simulink model "TestAsset14"  (R2018b)
settings: Solver=ode45  StartTime=0.0  StopTime=4  RelTol=1e-3  EnableMultiTasking=on
undefined symbols (not defined in the file): c1, c2, c3, c4, c5, c6, DiscIntNeverNeededParam, fdesignblkfcn, gcbh, Hydride, Metal, Nickel
libraries: powerlib x63, powerlib_extras x26, powerlib_meascontrol x25, simulink x5, simulink_extras x2, electricdrivelib x1
(part 2 of 3)

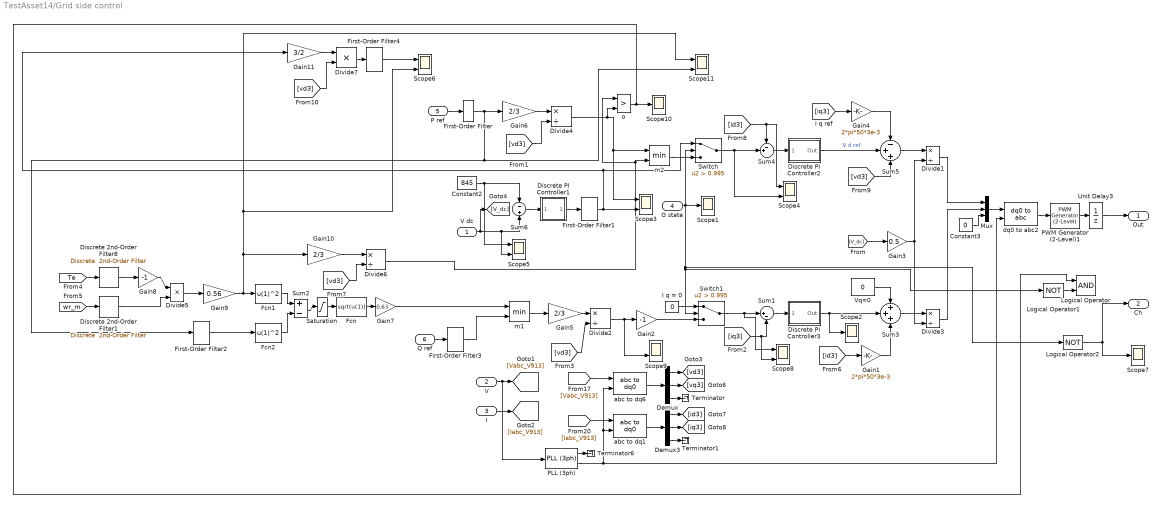
== system TestAsset14/Grid side control ==
  V dc : Inport
  V : Inport  Port=2
  I : Inport  Port=3
  G state : Inport  Port=4
  P ref : Inport  Port=5
  Q ref : Inport  Port=6
  Constant2 : Constant  Value=845
  Constant3 : Constant  Value=0
  Demux : Demux  Outputs=3
  Demux3 : Demux  Outputs=3
  Discrete PI Controller1 : Subsystem  DialogController=POWERSYS.PowerSysDialog  mask(Discrete PI Controller){Kp=10, Ki=60, Par_Limits=[500 -500], Init=0, Ts=20e-6}
      mask prompts: Kp "Proportional gain (Kp):"; Ki "Integral gain (Ki):"; Par_Limits "Output limits: [ Upper   Lower ]"; Init "Output initial value:"; Ts "Sample time:"
      mask help: This block implements a discrete PI controller.
      mask init:
      | UpperLimit=Par_Limits(1);
      | LowerLimit=Par_Limits(2);
      | power_initmask();
      mask Display: disp('PI');
  Discrete PI Controller2 : Subsystem  DialogController=POWERSYS.PowerSysDialog  mask(Discrete PI Controller){Kp=16, Ki=160, Par_Limits=[400 -400], Init=0, Ts=20e-6}
      mask prompts: Kp "Proportional gain (Kp):"; Ki "Integral gain (Ki):"; Par_Limits "Output limits: [ Upper   Lower ]"; Init "Output initial value:"; Ts "Sample time:"
      mask help: This block implements a discrete PI controller.
      mask init:
      | UpperLimit=Par_Limits(1);
      | LowerLimit=Par_Limits(2);
      | power_initmask();
      mask Display: disp('PI');
  Discrete PI Controller3 : Subsystem  DialogController=POWERSYS.PowerSysDialog  mask(Discrete PI Controller){Kp=16, Ki=160, Par_Limits=[400 -400], Init=0, Ts=20e-6}
      mask prompts: Kp "Proportional gain (Kp):"; Ki "Integral gain (Ki):"; Par_Limits "Output limits: [ Upper   Lower ]"; Init "Output initial value:"; Ts "Sample time:"
      mask help: This block implements a discrete PI controller.
      mask init:
      | UpperLimit=Par_Limits(1);
      | LowerLimit=Par_Limits(2);
      | power_initmask();
      mask Display: disp('PI');
  Discrete 2nd-Order Filter1 : powerlib_extras/Discrete  Control Blocks/Discrete  2nd-Order Filter  FilterType=Lowpass  Fo=50  Zeta=0.73  Ts=20e-6  Initialize=on  Vac_Init=[0.8 -25 60]*0  Vdc_Init=-183.8  PlotResponse=off  param1=[1 500 1]
  Discrete 2nd-Order Filter8 : powerlib_extras/Discrete  Control Blocks/Discrete  2nd-Order Filter  FilterType=Lowpass  Fo=50  Zeta=0.73  Ts=20e-6  Initialize=on  Vac_Init=[0.8 -25 60]*0  Vdc_Init=-183.8  PlotResponse=off  param1=[1 500 1]
  Divide{1..4,6} (5 alike) : Product  Inputs=*/
  Divide5 : Product  Inputs=**
  Divide7 : Product  Inputs=**
  Fcn : Fcn  Expr=sqrt(u(1))
  Fcn1 : Fcn  Expr=u(1)^2  SampleTime=20e-6
  Fcn2 : Fcn  Expr=u(1)^2  SampleTime=20e-6
  First-Order Filter{,1..4} (5 alike) : powerlib_meascontrol/Filters/First-Order Filter  FilterType=Lowpass  Tc=10e-3  Ts=20e-6  Initialize=on  Vac_Init=[0, 0, 60]  Vdc_Init=0  PlotResponse=off  FreqRange="[0,  200,  1]"
  Gain1 : Gain  Gain=2*pi*50*3e-3
  Gain10 : Gain  Gain=2/3
  Gain11 : Gain  Gain=3/2
  Gain2 : Gain  Gain=-1
  Gain3 : Gain  Gain=0.5
  Gain4 : Gain  Gain=2*pi*50*3e-3
  Gain5 : Gain  Gain=2/3
  Gain6 : Gain  Gain=2/3
  Gain7 : Gain  Gain=0.63
  Gain8 : Gain  Gain=-1
  Gain9 : Gain  Gain=0.56
  I q = 0 : Constant  Value=0
  Logical Operator : Logic  AllPortsSameDT=off  OutDataTypeStr=boolean  SampleTime=20e-6
  Logical Operator1 : Logic  Operator=NOT  AllPortsSameDT=off  OutDataTypeStr=boolean  SampleTime=20e-6
  Logical Operator2 : Logic  Operator=NOT  AllPortsSameDT=off  OutDataTypeStr=boolean  SampleTime=20e-6
  Mux : Mux  Inputs=3
  PLL (3ph) : powerlib_meascontrol/PLL/PLL (3ph)  Fmin=45  Par_Init=[0, 60]  ParK=[180, 3200, 1]  TcD=1e-4  MaxRateChangeFreq=12  FilterCutOffFreq=25  Ts=20e-6  AGC=on
  PWM Generator (2-Level)1 : powerlib_meascontrol/Pulse & Signal Generators/PWM Generator (2-Level)  ModulatorType=Three-phase bridge (6 pulses)  ModulatorMode=Unsynchronized  Fc=2000  Pc=90  nF=27  MinMax="[ -1  1 ]"  SamplingTechnique=Natural  ModulatingSignals=off  m=0.8  Freq=60  Phase=0  Ts=20e-6  ShowCarrierOutport=off
  Saturation : Saturate  UpperLimit=inf  LowerLimit=0
  Scope{1..2,7,10} (4 alike) : Scope
  Scope{3..6,8..9,11} (7 alike) : Scope  NumInputPorts=2
  Sum1 : Sum  Inputs=|+-
  Sum2 : Sum  Inputs=+-
  Sum3 : Sum  Inputs=+++
  Sum4 : Sum  Inputs=-+|
  Sum5 : Sum  Inputs=-++
  Sum6 : Sum  Inputs=-+
  Switch : Switch  Criteria=u2 > Threshold  Threshold=0.995
  Switch1 : Switch  Criteria=u2 > Threshold  Threshold=0.995
  Terminator : Terminator
  Terminator1 : Terminator
  Terminator6 : Terminator
  Unit Delay3 : UnitDelay  SampleTime=2e-05  HasFrameUpgradeWarning=on
  Vq=0 : Constant  Value=0
  abc to dq1 : powerlib_meascontrol/Transformations/abc to dq0  Alignment=90 degrees behind phase A axis
  abc to dq6 : powerlib_meascontrol/Transformations/abc to dq0  Alignment=90 degrees behind phase A axis
  dq0 to abc2 : powerlib_meascontrol/Transformations/dq0 to abc  Alignment=90 degrees behind phase A axis
  m1 : MinMax  Inputs=2  SampleTime=20e-6
  m2 : MinMax  Inputs=2  SampleTime=20e-6
  o : RelationalOperator  Operator=>  OutDataTypeStr=boolean  RndMeth=Nearest
  Out : Outport
  Ch : Outport  Port=2
  wires:
  abc to dq6/1 -> Demux/1
  Demux/1 -> [vd3]
  Demux/2 -> [vq3]
  abc to dq1/1 -> Demux3/1
  Demux3/1 -> [id3]
  Demux3/2 -> [iq3]
  [iq3] -> Scope8/2, Sum1/2
  Sum1/1 -> Discrete PI Controller3/1(Error)
  Discrete PI Controller3/1(Out) -> Scope2/1, Sum3/2
  Gain1/1 -> Sum3/3
  [id3] -> Gain1/1
  Sum3/1 -> Divide3/1
  Mux/1 -> dq0 to abc2/1
  [Vabc_V913] -> abc to dq6/1
  [Iabc_V913] -> abc to dq1/1
  dq0 to abc2/1 -> PWM Generator (2-Level)1/1
  Constant3/1 -> Mux/3
  PLL (3ph)/2 -> dq0 to abc2/2, abc to dq1/2, abc to dq6/2
  V/1 -> PLL (3ph)/1, [Vabc_V913]
  Discrete PI Controller2/1(Out) -> Sum5/2  "V d ref"
  [vd3] -> Sum5/3
  Sum4/1 -> Discrete PI Controller2/1(Error)
  Gain4/1 -> Sum5/1
  Sum6/1 -> Discrete PI Controller1/1(Error)
  Sum5/1 -> Divide1/1
  I/1 -> [Iabc_V913]
  [iq3] -> Gain4/1
  Demux/3 -> Terminator/1
  Demux3/3 -> Terminator1/1
  Vq=0/1 -> Sum3/1
  Divide1/1 -> Mux/1
  Divide3/1 -> Mux/2
  Gain3/1 -> Divide1/2, Divide3/2
  [V_dc] -> Gain3/1
  PLL (3ph)/1 -> Terminator6/1
  [id3] -> Scope4/1, Sum4/1
  Switch1/1 -> Scope8/1, Sum1/1
  G state/1 -> Switch/2, Scope1/1, Logical Operator2/1, Logical Operator1/1, Switch1/2
  Divide4/1 -> o/2, m2/1, Scope3/1
  Switch/1 -> Scope4/2, Sum4/2
  [vd3] -> Divide4/2
  Gain6/1 -> Divide4/1
  m2/1 -> Switch/3
  Discrete PI Controller1/1(Out) -> First-Order Filter1/1
  I q = 0/1 -> Switch1/1
  [vd3] -> Divide2/2
  Gain5/1 -> Divide2/1
  Saturation/1 -> Fcn/1
  PWM Generator (2-Level)1/1 -> Unit Delay3/1
  Unit Delay3/1 -> Out/1
  Logical Operator2/1 -> Ch/1, Scope7/1
  o/1 -> Scope10/1, Logical Operator/1
  Logical Operator1/1 -> Logical Operator/2
  Gain2/1 -> Switch1/3
  Gain8/1 -> Divide5/1
  Discrete 2nd-Order Filter1/1 -> Divide5/2
  Divide5/1 -> Gain9/1
  V dc/1 -> Scope5/2, Sum6/2, [V_dc]
  Discrete 2nd-Order Filter8/1 -> Gain8/1
  [Te] -> Discrete 2nd-Order Filter8/1
  Gain9/1 -> Scope11/1, Scope6/2, Gain10/1, Fcn1/1
  [wr_m] -> Discrete 2nd-Order Filter1/1
  Fcn1/1 -> Sum2/1
  Fcn2/1 -> Sum2/2
  Sum2/1 -> Saturation/1
  Divide2/1 -> Scope9/2, Gain2/1
  First-Order Filter2/1 -> Fcn2/1
  First-Order Filter3/1 -> m1/2
  Q ref/1 -> First-Order Filter3/1
  Gain7/1 -> m1/1
  Fcn/1 -> Gain7/1
  Constant2/1 -> Sum6/1, Scope5/1
  [vd3] -> Divide7/2
  Gain11/1 -> Divide7/1
  Divide7/1 -> First-Order Filter4/1
  First-Order Filter4/1 -> Scope6/1
  First-Order Filter1/1 -> Gain11/1, Switch/1, Scope3/2
  m1/1 -> Gain5/1
  P ref/1 -> First-Order Filter/1
  First-Order Filter/1 -> Scope11/2, First-Order Filter2/1, Gain6/1
  Gain10/1 -> Divide6/1
  [vd3] -> Divide6/2
  Divide6/1 -> o/1, m2/2

== system TestAsset14/LC Filter ==
  "2 mH " : powerlib/Elements/Three-Phase Series RLC Branch  LConnTagsString=A|B|C  RConnTagsString=A|B|C  BranchType=L  Resistance=1.0  Inductance=3e-3  Capacitance=1.0  Measurements=None
  Ground : powerlib/Elements/Ground  LConnTagsString=a
  Ground1 : powerlib/Elements/Ground  LConnTagsString=a
  Ground2 : powerlib/Elements/Ground  LConnTagsString=a
  Three-Phase Series RLC Branch : powerlib/Elements/Three-Phase Series RLC Branch  LConnTagsString=A|B|C  RConnTagsString=A|B|C  BranchType=C  Resistance=.1  Inductance=1e-3  Capacitance=100e-6  Measurements=None
  A : PMIOPort  Side=Left
  B : PMIOPort  Port=2  Side=Left
  C : PMIOPort  Port=3  Side=Left
  "A " : PMIOPort  Port=4  Side=Right
  "B " : PMIOPort  Port=5  Side=Right
  "C " : PMIOPort  Port=6  Side=Right
  connections:
  B/RConn1 -- "2 mH "/LConn2
  A/RConn1 -- "2 mH "/LConn1
  C/RConn1 -- "2 mH "/LConn3
  "2 mH "/RConn1 -- "A "/RConn1 -- Three-Phase Series RLC Branch/LConn1
  "2 mH "/RConn2 -- "B "/RConn1 -- Three-Phase Series RLC Branch/LConn2
  "2 mH "/RConn3 -- "C "/RConn1 -- Three-Phase Series RLC Branch/LConn3
  Ground/LConn1 -- Three-Phase Series RLC Branch/RConn1
  Ground1/LConn1 -- Three-Phase Series RLC Branch/RConn2
  Ground2/LConn1 -- Three-Phase Series RLC Branch/RConn3

== system TestAsset14/LC Filter1 ==
  "2 mH " : powerlib/Elements/Three-Phase Series RLC Branch  LConnTagsString=A|B|C  RConnTagsString=A|B|C  BranchType=L  Resistance=0  Inductance=3e-3  Capacitance=inf  Measurements=None
  3 kvar : powerlib/Elements/Three-Phase Series RLC Load  LConnTagsString=A|B|C  Configuration=Y (grounded)  NominalVoltage=480  NominalFrequency=50  ActivePower=0  InductivePower=0  CapacitivePower=3e3  Measurements=None  LoadType=constant Z
  A : PMIOPort  Side=Left
  B : PMIOPort  Port=2  Side=Left
  C : PMIOPort  Port=3  Side=Left
  "A " : PMIOPort  Port=4  Side=Right
  "B " : PMIOPort  Port=5  Side=Right
  "C " : PMIOPort  Port=6  Side=Right
  connections:
  C/RConn1 -- "2 mH "/LConn3
  "2 mH "/LConn2 -- B/RConn1
  "2 mH "/LConn1 -- A/RConn1
  "A "/RConn1 -- 3 kvar/LConn1 -- "2 mH "/RConn1
  3 kvar/LConn3 -- "2 mH "/RConn3 -- "C "/RConn1
  3 kvar/LConn2 -- "2 mH "/RConn2 -- "B "/RConn1

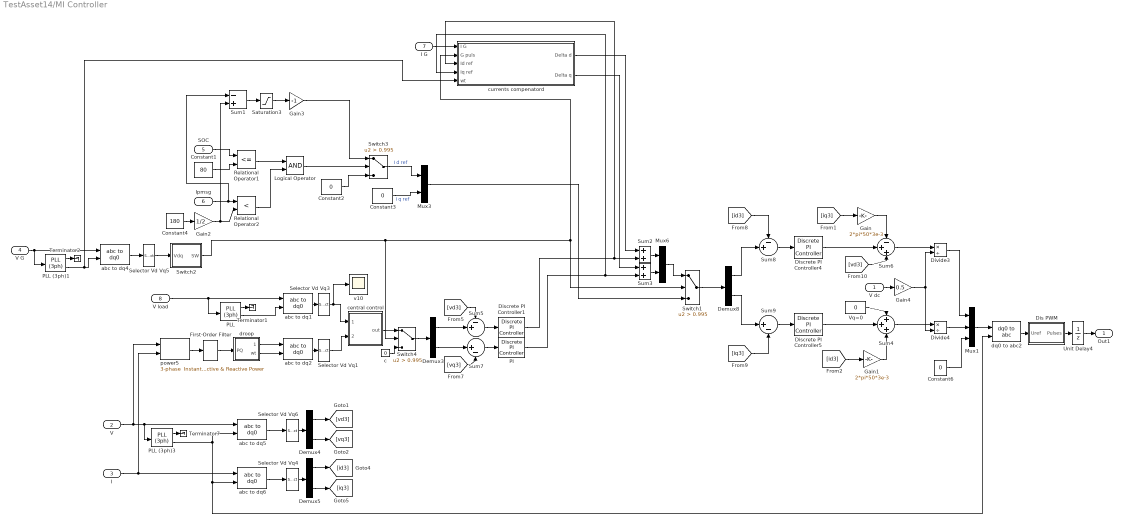
== system TestAsset14/MI Controller ==
  V dc : Inport
  V : Inport  Port=2
  I : Inport  Port=3
  V G : Inport  Port=4
  SOC : Inport  Port=5
  Ipmsg : Inport  Port=6
  I G : Inport  Port=7
  V load : Inport  Port=8
  Constant1 : Constant  Value=80
  Constant2 : Constant  Value=0
  Constant3 : Constant  Value=0
  Constant4 : Constant  Value=180
  Constant6 : Constant  Value=0
  Demux{3..5,8} (4 alike) : Demux  Outputs=2
  Dis PWM : Subsystem  AncestorBlock=|  DialogController=POWERSYS.PowerSysDialog  mask(Discrete PWM Generator){GeneratorMode=3-arm  bridge (6 pulses), Fc=4000, Ts=20e-6, Internal=off, mIndex=0.4, Freq=60, Phase=0}
      | powerlib_extras/Discrete 
      | Control Blocks/Discrete
      | PWM Generator
      mask prompts: GeneratorMode "Generator Mode"; Fc "Carrier frequency (Hz):"; Ts "Sample time:"; Internal "Internal generation of modulating signal(s)"; mIndex "Modulation index  (0<m<1) :"; Freq "Frequency of output voltage (Hz)"; Phase "Phase of output voltage (degrees)"
      mask help:
      | This discrete block generates pulses for carrier-based PWM (Pulse Width Modulation), self-commutated IGBTs,GTOs or FETs bridges.
      |
      | Depending on the number of bridge arms selected in the "Generator Mode" parameter, the block can be used either for single-phase or three-phase PWM control.
      mask init:
      | powericon('psbcallbacks',gcb,'Discrete PWM Generator');
      | if Freq==0
      |     Phase=90;
      | end
      | switch GeneratorMode
      | case 1,
      |     Internal_Phase=0;
      |    Signal_PortWidth=1;
      |    Select1_Elements=[1 2];
      |    Select1_PortWidth=2;
      |    Select3_Elements=[1 2];
      |    Select3_PortWidth=4;
      | case 2,
      |     Internal_Phase=0;
      |     Signal_PortWidth=1;
      |     Select1_Elements=[1 2];
      |     Select1_PortWidth=2;
      |     Select3_Elements=[1 2 3 4];
      |     Select3_PortWidth=4;
      | case 3,
      |     Internal_Phase=[0 -2*pi/3 2*pi/3];
      |     Signal_PortWidth=3;
      |     Select1_Elements=[1 4 2 5 3 6];
      |     Select1_PortWidth=6;
      |    Select3_Elements=[1 2 3 4 5 6];
      |    Select3_PortWidth=12;
      | case 4,
      |     Internal_Phase=[0 -2*pi/3 2*pi/3];
      |     Signal_PortWidth=3;
      |     Select1_Elements=[1 4 2 5 3 6];
      |     Select1_PortWidth=6;
      |    Select3_Elements=[1 2 3 4 5 6 7 8 9 10 11 12];
      |    Select3_PortWidth=12;
      | end
      | power_initmask();
      mask Help:
      | The output pulses are a vector (with values=0 or 1). Depending on the selected "Generator Mode", the output vector contains:
      | For a 1-arm  bridge: Two pulses. Pulse 1 is for the upper switch and pulse 2 is for the lower switch.
      | For a 2-arm  bridge: Four pulses. Pulses 1 and 3 are respectively for the upper switches of the first and second arm. Pulses 2 and 4 are for the lower switches.
      | For a 3-arm  bridge: Six pulses. Pulses 1,3 and 5 are respectively for the upper switches of the first,second and third arm. Pulses 2,4 and 6 are for the lower switches.
      | For double 3-arm bridges: Twelve pulses.The first six pulses (pulses 1 to 6) must be sent to the first 3-arm bridge and the last six (pulses 7 to 12) to the second 3-arm bridge.
      | 
      | By selecting "Internal generation" you can can control the modulation index m, frequency and phase of the output voltage  from the internal parameters (m, Freq and Phase). Otherwise, external signals are used for pulse generation. The width of the input vector must be 1 for single phase bridges ( 1-arm or 2-arm)  and 3 for 3-phase bridges  (single or double bridge).
      mask TypeOptions GeneratorMode: 1-arm  bridge (2 pulses) | 2-arm  bridge (4 pulses) | 3-arm  bridge (6 pulses) | Double 3-arm  bridges (12 pulses)
      mask Callback Internal: powericon('psbcallbacks',gcb,'Discrete PWM Generator',[]);
  Discrete PI Controller1 : powerlib_extras/Discrete  Control Blocks/Discrete PI Controller  Kp=8  Ki=20  Par_Limits=[460 -460]  Init=0  Ts=20e-6
  Discrete PI Controller4 : powerlib_extras/Discrete  Control Blocks/Discrete PI Controller  Kp=2  Ki=40  Par_Limits=[400 -400]  Init=0.1  Ts=20e-6
  Discrete PI Controller5 : powerlib_extras/Discrete  Control Blocks/Discrete PI Controller  Kp=2  Ki=40  Par_Limits=[400 -400]  Init=0.1  Ts=20e-6
  Divide3 : Product  Inputs=*/
  Divide4 : Product  Inputs=*/
  First-Order Filter : powerlib_meascontrol/Filters/First-Order Filter  FilterType=Lowpass  Tc=1e-3  Ts=0  Initialize=on  Vac_Init=[0, 0, 50]  Vdc_Init=0  PlotResponse=off  FreqRange="[0,  200,  1]"
  Gain : Gain  Gain=2*pi*50*3e-3
  Gain1 : Gain  Gain=2*pi*50*3e-3
  Gain2 : Gain  Gain=1/2
  Gain3 : Gain  Gain=-1
  Gain4 : Gain  Gain=0.5
  Logical Operator : Logic  AllPortsSameDT=off  OutDataTypeStr=boolean
  Mux1 : Mux  Inputs=3
  Mux3 : Mux  Inputs=2
  Mux6 : Mux  Inputs=2
  "PI " : powerlib_extras/Discrete  Control Blocks/Discrete PI Controller  Kp=8  Ki=20  Par_Limits=[400 -400]  Init=0  Ts=20e-6
  "PLL " : powerlib_meascontrol/PLL/PLL (3ph)  Fmin=45  Par_Init=[0, 50]  ParK=[180, 3200, 1]  TcD=1e-4  MaxRateChangeFreq=12  FilterCutOffFreq=25  Ts=2e-05  AGC=on
  PLL (3ph)1 : powerlib_meascontrol/PLL/PLL (3ph)  Fmin=45  Par_Init=[0, 50]  ParK=[180, 3200, 1]  TcD=1e-4  MaxRateChangeFreq=12  FilterCutOffFreq=25  Ts=2e-05  AGC=on
  PLL (3ph)3 : powerlib_meascontrol/PLL/PLL (3ph)  Fmin=45  Par_Init=[0, 50]  ParK=[180, 3200, 1]  TcD=1e-4  MaxRateChangeFreq=12  FilterCutOffFreq=25  Ts=2e-05  AGC=on
  Relational Operator1 : RelationalOperator  Operator=<=  RndMeth=Nearest  InputSameDT=on
  Relational Operator2 : RelationalOperator  Operator=<  RndMeth=Nearest  InputSameDT=on
  Saturation3 : Saturate  UpperLimit=90  LowerLimit=0  SampleTime=2e-05
  Selector Vd Vq{1,3..6} (5 alike) : Selector  InputPortWidth=3  IndexOptions=Index vector (dialog)  Indices=[1 2]  OutputSizes=1
  Sum1 : Sum  Inputs=-+
  Sum2 : Sum
  Sum3 : Sum
  Sum4 : Sum  Inputs=+++
  Sum5 : Sum  Inputs=-+|
  Sum6 : Sum  Inputs=-++
  Sum7 : Sum  Inputs=|+-
  Sum8 : Sum  Inputs=-+|
  Sum9 : Sum  Inputs=|+-
  Switch1 : Switch  Criteria=u2 > Threshold  Threshold=0.995
  Switch2 : Subsystem
  Switch3 : Switch  Criteria=u2 > Threshold  Threshold=0.995
  Switch4 : Switch  Criteria=u2 > Threshold  Threshold=0.995
  Terminator1 : Terminator
  Terminator2 : Terminator
  Terminator7 : Terminator
  Unit Delay4 : UnitDelay  SampleTime=20e-6  HasFrameUpgradeWarning=on
  Vq=0 : Constant  Value=0
  abc to dq{1..2,4..6} (5 alike) : powerlib_meascontrol/Transformations/abc to dq0  Alignment=90 degrees behind phase A axis
  c : Constant  Value=0
  central control : Subsystem
  currents compenatord : Subsystem
  dq0 to abc2 : powerlib_meascontrol/Transformations/dq0 to abc  Alignment=90 degrees behind phase A axis
  droop : Subsystem
  power5 : powerlib_extras/Measurements/3-phase  Instantaneous  Active & Reactive Power
  v10 : Scope
  Out1 : Outport
  wires:
  Demux3/2 -> Sum7/1
  Demux3/1 -> Sum5/2
  [vq3] -> Sum7/2
  Sum5/1 -> Discrete PI Controller1/1
  Sum7/1 -> "PI "/1
  [id3] -> Sum8/1
  [iq3] -> Sum9/2
  Sum8/1 -> Discrete PI Controller4/1
  Sum9/1 -> Discrete PI Controller5/1
  Discrete PI Controller4/1 -> Sum6/2
  Discrete PI Controller5/1 -> Sum4/2
  Constant6/1 -> Mux1/3
  Mux1/1 -> dq0 to abc2/1
  dq0 to abc2/1 -> Dis PWM/1(Uref)
  Sum6/1 -> Divide3/1
  [id3] -> Gain1/1
  [iq3] -> Gain/1
  Gain1/1 -> Sum4/3
  Gain/1 -> Sum6/1
  [vd3] -> Sum5/1
  Sum4/1 -> Divide4/1
  Divide3/1 -> Mux1/1
  Divide4/1 -> Mux1/2
  V dc/1 -> Gain4/1
  Gain4/1 -> Divide4/2, Divide3/2
  I/1 -> abc to dq6/1, power5/2
  Demux4/2 -> [vq3]
  abc to dq5/1 -> Selector Vd Vq6/1
  Demux5/2 -> [iq3]
  Demux5/1 -> [id3]
  Selector Vd Vq4/1 -> Demux5/1
  abc to dq6/1 -> Selector Vd Vq4/1
  V/1 -> abc to dq5/1, PLL (3ph)3/1, power5/1
  Demux4/1 -> [vd3]
  [vd3] -> Sum6/3
  Vq=0/1 -> Sum4/1
  First-Order Filter/1 -> droop/1(PQ)
  droop/1(Vabc) -> abc to dq2/1
  droop/2(wt) -> abc to dq2/2
  abc to dq2/1 -> Selector Vd Vq1/1
  Selector Vd Vq6/1 -> Demux4/1
  PLL (3ph)3/2 -> abc to dq6/2, dq0 to abc2/2, abc to dq5/2
  PLL (3ph)3/1 -> Terminator7/1
  Constant3/1 -> Mux3/2  "I q ref"
  Switch3/1 -> Mux3/1  "I d ref"
  abc to dq4/1 -> Selector Vd Vq5/1
  V G/1 -> abc to dq4/1, PLL (3ph)1/1
  Constant2/1 -> Switch3/3
  SOC/1 -> Relational Operator1/1
  Constant1/1 -> Relational Operator1/2
  Selector Vd Vq5/1 -> Switch2/1(Vdq)
  Gain3/1 -> Switch3/1
  PLL (3ph)1/1 -> Terminator2/1
  Relational Operator1/1 -> Logical Operator/1
  Ipmsg/1 -> Sum1/1, Relational Operator2/1
  Gain2/1 -> Relational Operator2/2, Sum1/2
  Constant4/1 -> Gain2/1
  Relational Operator2/1 -> Logical Operator/2
  Sum1/1 -> Saturation3/1
  Saturation3/1 -> Gain3/1
  Demux8/1 -> Sum8/2
  Demux8/2 -> Sum9/1
  Logical Operator/1 -> Switch3/2
  Discrete PI Controller1/1 -> currents compenatord/3(Id ref), Sum2/2
  "PI "/1 -> currents compenatord/4(Iq ref), Sum3/2
  Switch1/1 -> Demux8/1
  Mux6/1 -> Switch1/1
  PLL (3ph)1/2 -> currents compenatord/5(wt), abc to dq4/2
  Sum2/1 -> Mux6/1
  Sum3/1 -> Mux6/2
  I G/1 -> currents compenatord/1(I G)
  currents compenatord/1(Delta d) -> Sum2/1
  currents compenatord/2(Delta q) -> Sum3/1
  Mux3/1 -> Switch1/3
  Dis PWM/1(Pulses) -> Unit Delay4/1
  Unit Delay4/1 -> Out1/1
  power5/1 -> First-Order Filter/1
  abc to dq1/1 -> Selector Vd Vq3/1
  V load/1 -> "PLL "/1, abc to dq1/1
  "PLL "/2 -> abc to dq1/2
  "PLL "/1 -> Terminator1/1
  Switch4/1 -> Demux3/1
  Switch2/1(SW) -> Switch4/2, currents compenatord/2(G puls), Switch1/2
  Selector Vd Vq3/1 -> central control/1(Vdq_load), v10/1
  Selector Vd Vq1/1 -> central control/2(Vdq_droop)
  c/1 -> Switch4/3
  central control/1(out) -> Switch4/1

== system TestAsset14/P load ==
  L : Inport
  S2 : Fcn  Expr=sqrt(u(1)^2+u(2)^2)
  Selector Vd Vq1 : Selector  InputPortWidth=2  IndexOptions=Index vector (dialog)  Indices=[2]  OutputSizes=1
  Selector Vd Vq2 : Selector  InputPortWidth=2  IndexOptions=Index vector (dialog)  Indices=[1]  OutputSizes=1
  P : Outport
  Q : Outport  Port=2
  S : Outport  Port=3
  wires:
  L/1 -> Selector Vd Vq1/1, S2/1, Selector Vd Vq2/1
  Selector Vd Vq2/1 -> P/1
  Selector Vd Vq1/1 -> Q/1
  S2/1 -> S/1

== system TestAsset14/Pitch_angle-controller ==
  wr : Inport
  0-pitch_max : Saturate  UpperLimit=45  LowerLimit=0
  Constant2 : Constant  Value=2
  "Rate Limiter   " : RateLimiter  RisingSlewLimit=2  FallingSlewLimit=-2
  Sum : Sum  Inputs=|+-  SaturateOnIntegerOverflow=on
  genertaor terminal6 : Scope  NumInputPorts=2
  pitch_gain : Gain  Gain=500  SaturateOnIntegerOverflow=on  OutDataTypeStr=Inherit: Same as input  ParamDataTypeStr=Inherit: Same as input
  Pitch_angle : Outport
  wires:
  "Rate Limiter   "/1 -> Pitch_angle/1, genertaor terminal6/1
  pitch_gain/1 -> 0-pitch_max/1
  Sum/1 -> pitch_gain/1
  Constant2/1 -> Sum/2
  0-pitch_max/1 -> "Rate Limiter   "/1, genertaor terminal6/2
  wr/1 -> Sum/1

== system TestAsset14/Wind Turbine model ==
  Generator speed (pu) : Inport
  Pitch angle (deg) : Inport  Port=2
  Wind speed (m/s) : Inport  Port=3
  1/cp_nom : Gain  Gain=1/cp_nom  SaturateOnIntegerOverflow=on  OutDataTypeStr=Inherit: Same as input  ParamDataTypeStr=Inherit: Same as input
  1/wind_base : Gain  Gain=1/wind_base  SaturateOnIntegerOverflow=on  OutDataTypeStr=Inherit: Same as input  ParamDataTypeStr=Inherit: Same as input
  Avoid division by zero : Saturate  UpperLimit=1e6  LowerLimit=1e-6
  "Avoid division by zero " : Saturate  UpperLimit=1e6  LowerLimit=1e-6
  Gain : Gain  Gain=-1  SaturateOnIntegerOverflow=on  OutDataTypeStr=Inherit: Same as input  ParamDataTypeStr=Inherit: Same as input
  Product : Product  Inputs=/*  SaturateOnIntegerOverflow=on  OutDataTypeStr=Inherit: Same as first input
  "Product " : Product  SaturateOnIntegerOverflow=on  OutDataTypeStr=Inherit: Same as first input
  Product2 : Product  Inputs=*/  InputSameDT=on  SaturateOnIntegerOverflow=on  OutDataTypeStr=Inherit: Same as first input
  Saturation1 : Saturate  UpperLimit=inf  LowerLimit=1e-6
  Scope : Scope
  cp(lambda,beta) : Subsystem
  lambda_nom : Gain  Gain=lambda_nom  SaturateOnIntegerOverflow=on  OutDataTypeStr=Inherit: Same as input  ParamDataTypeStr=Inherit: Same as input
  pu->pu : Gain  Gain=P_wind_base*Pnom/Pelec_base  SaturateOnIntegerOverflow=on  OutDataTypeStr=Inherit: Same as input  ParamDataTypeStr=Inherit: Same as input
  "pu->pu " : Gain  Gain=1/speed_nom  SaturateOnIntegerOverflow=on  OutDataTypeStr=Inherit: Same as input  ParamDataTypeStr=Inherit: Same as input
  wind_speed^3 : Fcn  Expr=u(1)^3
  Tm (pu) : Outport
  wires:
  Pitch angle (deg)/1 -> cp(lambda,beta)/2(beta)
  pu->pu/1 -> Product2/1
  cp(lambda,beta)/1(cp) -> 1/cp_nom/1
  wind_speed^3/1 -> "Product "/1  "Pwind_pu"
  Product2/1 -> Gain/1
  Avoid division by zero/1 -> Product2/2
  Wind speed (m/s)/1 -> 1/wind_base/1
  Gain/1 -> Tm (pu)/1
  Generator speed (pu)/1 -> Avoid division by zero/1, "pu->pu "/1
  "Product "/1 -> pu->pu/1  "Pm_pu"
  lambda_nom/1 -> Saturation1/1  "lambda"
  1/cp_nom/1 -> "Product "/2  "cp_pu"
  Saturation1/1 -> cp(lambda,beta)/1(lambda), Scope/1
  Product/1 -> lambda_nom/1  "lambda_pu"
  1/wind_base/1 -> wind_speed^3/1, "Avoid division by zero "/1  "wind_speed_pu"
  "Avoid division by zero "/1 -> Product/1
  "pu->pu "/1 -> Product/2

== system TestAsset14/Wind-MPPT ==
  wm : Inport
  Ia : Inport  Port=2
  Vd : Inport  Port=3
  Avoid division by zero : Saturate  UpperLimit=1e6  LowerLimit=1e-6
  Base Torque1 : Product  Inputs=*/  RndMeth=Zero
  Discrete 1st-Order Filter2 : powerlib_extras/Discrete  Control Blocks/Discrete 1st-Order Filter  FilterType=Lowpass  Tc=200e-3  Ts=20e-6  Initialize=off  Vac_Init=[0.8 -25 60]  Vdc_Init=-0.4  PlotResponse=off  param1=[1 500 0.1]
  Discrete PI Controller2 : Subsystem  DialogController=POWERSYS.PowerSysDialog  mask(Discrete PI Controller){Kp=0.25, Ki=10, Par_Limits=[1 0], Init=0.2, Ts=2e-05}
      mask prompts: Kp "Proportional gain (Kp):"; Ki "Integral gain (Ki):"; Par_Limits "Output limits: [ Upper   Lower ]"; Init "Output initial value:"; Ts "Sample time:"
      mask help: This block implements a discrete PI controller.
      mask init:
      | UpperLimit=Par_Limits(1);
      | LowerLimit=Par_Limits(2);
      | power_initmask();
      mask Help: This block is part of a subset of blocks in the Extras library that does not have documentation associated with it, other than the block mask description.
      mask Display: disp('PI');
  Product1 : Product  RndMeth=Zero
  Pulse Generator : Subsystem
  Subtract : Sum  Inputs=+-
  Torque reference 1 : Subsystem
  Unit Delay3 : UnitDelay  SampleTime=-1  HasFrameUpgradeWarning=on
  Unit Delay4 : UnitDelay  SampleTime=2e-05  HasFrameUpgradeWarning=on
  p : Outport
  wires:
  Unit Delay3/1 -> Subtract/2
  Base Torque1/1 -> Discrete 1st-Order Filter2/1
  Discrete 1st-Order Filter2/1 -> Subtract/1
  Ia/1 -> Unit Delay3/1
  Vd/1 -> Avoid division by zero/1
  wm/1 -> Product1/2, Torque reference 1/1(wm)
  Torque reference 1/1(Tref) -> Product1/1
  Avoid division by zero/1 -> Base Torque1/2
  Product1/1 -> Base Torque1/1
  Unit Delay4/1 -> p/1
  Discrete PI Controller2/1(Out) -> Pulse Generator/1(Duty_Cycle)
  Pulse Generator/1(Pulse) -> Unit Delay4/1
  Subtract/1 -> Discrete PI Controller2/1(Error)

== system TestAsset14/300 kw Wind Turbine and Drive Train1/Drive Train ==
  note: Wind turbine drive train based on a 2-masse model
  note: Turbine
  note: Shaft
  T_wt (pu) : Inport
  Generator speed (pu) : Inport  Port=2
  1_2H_WT : Gain  Gain=1/(2*H_WT)  SaturateOnIntegerOverflow=on  OutDataTypeStr=Inherit: Same as input  ParamDataTypeStr=Inherit: Same as input
  Discrete-Time Integrator : DiscreteIntegrator  InitialCondition=w_wt0  SampleTime=Ts  ICPrevOutput=DiscIntNeverNeededParam  ICPrevScaledInput=DiscIntNeverNeededParam
  Discrete-Time Integrator1 : DiscreteIntegrator  InitialCondition=torque0/Ksh  SampleTime=Ts  ICPrevOutput=DiscIntNeverNeededParam  ICPrevScaledInput=DiscIntNeverNeededParam
  Mutual damping : Gain  Gain=D_mutual  SaturateOnIntegerOverflow=on  OutDataTypeStr=Inherit: Same as input  ParamDataTypeStr=Inherit: Same as input
  Stiffness : Gain  Gain=Ksh  SaturateOnIntegerOverflow=on  OutDataTypeStr=Inherit: Same as input  ParamDataTypeStr=Inherit: Same as input
  Sum : Sum  Inputs=+-  InputSameDT=on  SaturateOnIntegerOverflow=on  OutDataTypeStr=Inherit: Same as first input
  Sum1 : Sum  Inputs=+-  InputSameDT=on  SaturateOnIntegerOverflow=on  OutDataTypeStr=Inherit: Same as first input
  Sum2 : Sum  InputSameDT=on  SaturateOnIntegerOverflow=on  OutDataTypeStr=Inherit: Same as first input
  shaft_base_speed(rad/s) : Gain  Gain=shaft_base_speed  SaturateOnIntegerOverflow=on  OutDataTypeStr=Inherit: Same as input  ParamDataTypeStr=Inherit: Same as input
  W_wt (pu) : Outport
  T_shaft (pu) : Outport  Port=2
  wires:
  T_wt (pu)/1 -> Sum/1
  Sum2/1 -> T_shaft (pu)/1, Sum/2
  Mutual damping/1 -> Sum2/2
  Sum1/1 -> Mutual damping/1, shaft_base_speed(rad/s)/1
  Generator speed (pu)/1 -> Sum1/2
  Discrete-Time Integrator/1 -> W_wt (pu)/1, Sum1/1
  1_2H_WT/1 -> Discrete-Time Integrator/1
  Sum/1 -> 1_2H_WT/1
  Stiffness/1 -> Sum2/1
  Discrete-Time Integrator1/1 -> Stiffness/1
  shaft_base_speed(rad/s)/1 -> Discrete-Time Integrator1/1

== system TestAsset14/300 kw Wind Turbine and Drive Train1/Wind Turbine ==
  W_wt (pu) : Inport
  Pitch angle (deg) : Inport  Port=2
  Wind speed (m/s) : Inport  Port=3
  ->pu : Gain  Gain=1/Pmec
  Avoid div. by zero : Saturate  UpperLimit=inf  LowerLimit=eps
  "Avoid div. by zero " : Saturate  UpperLimit=inf  LowerLimit=eps
  Fcn1 : Fcn  Expr=K1*u[2]/u[1]
  Fcn2 : Fcn  Expr=c1*(c6*u[1] + (-c4 - c3*(2.5 + u[2]) + c2*(1/(u[1] + c7*(2.5 + u[2])) -c8/(1 + (2.5 + u[2])^3)))/exp(c5*(1/(u[1] + c7*(2.5 + u[2])) - c8/(1 + (2.5 + u[2])^3))))
  "K2*Cp*wind^3 " : Fcn  Expr=K2*u[1]^3*u[2]
  Mux : Mux  Inputs=2
  Mux1 : Mux  Inputs=2
  Mux2 : Mux  Inputs=2
  Product2 : Product  Inputs=*/  InputSameDT=on  SaturateOnIntegerOverflow=on  OutDataTypeStr=Inherit: Same as first input
  Tt (pu) : Outport
  wires:
  ->pu/1 -> Product2/1  "power_pu"
  Product2/1 -> Tt (pu)/1
  Wind speed (m/s)/1 -> Avoid div. by zero/1
  Fcn1/1 -> Mux1/1  "lambda"
  Mux1/1 -> Fcn2/1
  Mux/1 -> Fcn1/1
  Fcn2/1 -> Mux2/2  "Cp"
  Mux2/1 -> "K2*Cp*wind^3 "/1
  Pitch angle (deg)/1 -> Mux1/2
  W_wt (pu)/1 -> "Avoid div. by zero "/1
  Avoid div. by zero/1 -> Mux2/1, Mux/1
  "Avoid div. by zero "/1 -> Mux/2, Product2/2
  "K2*Cp*wind^3 "/1 -> ->pu/1

== system TestAsset14/Battery//electrolyzer controller/Discrete PI Controller ==
  Error : Inport
  Discrete-Time Integrator : DiscreteIntegrator  InitialCondition=Init  SampleTime=Ts  LimitOutput=on  UpperSaturationLimit=UpperLimit  LowerSaturationLimit=LowerLimit  ICPrevOutput=DiscIntNeverNeededParam  ICPrevScaledInput=DiscIntNeverNeededParam
  Kp4 : Gain  Gain=Kp  SaturateOnIntegerOverflow=on  OutDataTypeStr=Inherit: Same as input  ParamDataTypeStr=Inherit: Same as input
  Kp5 : Gain  Gain=Ki  SaturateOnIntegerOverflow=on  OutDataTypeStr=Inherit: Same as input  ParamDataTypeStr=Inherit: Same as input
  Saturation2 : Saturate  UpperLimit=UpperLimit  LowerLimit=LowerLimit
  Sum6 : Sum  InputSameDT=on  SaturateOnIntegerOverflow=on  OutDataTypeStr=Inherit: Same as first input
  Out : Outport  InitialOutput=0
  wires:
  Saturation2/1 -> Out/1
  Discrete-Time Integrator/1 -> Sum6/2
  Kp4/1 -> Sum6/1
  Kp5/1 -> Discrete-Time Integrator/1
  Sum6/1 -> Saturation2/1
  Error/1 -> Kp5/1, Kp4/1

== system TestAsset14/Battery//electrolyzer controller/Discrete PI Controller1 ==
  Error : Inport
  Discrete-Time Integrator : DiscreteIntegrator  InitialCondition=Init  SampleTime=Ts  LimitOutput=on  UpperSaturationLimit=UpperLimit  LowerSaturationLimit=LowerLimit  ICPrevOutput=DiscIntNeverNeededParam  ICPrevScaledInput=DiscIntNeverNeededParam
  Kp4 : Gain  Gain=Kp  SaturateOnIntegerOverflow=on  OutDataTypeStr=Inherit: Same as input  ParamDataTypeStr=Inherit: Same as input
  Kp5 : Gain  Gain=Ki  SaturateOnIntegerOverflow=on  OutDataTypeStr=Inherit: Same as input  ParamDataTypeStr=Inherit: Same as input
  Saturation2 : Saturate  UpperLimit=UpperLimit  LowerLimit=LowerLimit
  Sum6 : Sum  InputSameDT=on  SaturateOnIntegerOverflow=on  OutDataTypeStr=Inherit: Same as first input
  Out : Outport  InitialOutput=0
  wires:
  Saturation2/1 -> Out/1
  Discrete-Time Integrator/1 -> Sum6/2
  Kp4/1 -> Sum6/1
  Kp5/1 -> Discrete-Time Integrator/1
  Sum6/1 -> Saturation2/1
  Error/1 -> Kp5/1, Kp4/1

== system TestAsset14/Battery//electrolyzer controller/Ramp_generator ==
  note: Carrier Freq
  Constant3 : Constant
  Discrete-Time Integrator1 : DiscreteIntegrator  ExternalReset=rising  SampleTime=20e-6  ICPrevOutput=DiscIntNeverNeededParam  ICPrevScaledInput=DiscIntNeverNeededParam
  Relational Operator1 : RelationalOperator  RndMeth=Nearest  InputSameDT=on
  Unit Delay1 : UnitDelay  SampleTime=20e-6  HasFrameUpgradeWarning=on
  fc : Constant  Value=10000
  ramp_out : Outport
  wires:
  Unit Delay1/1 -> Discrete-Time Integrator1/2
  Relational Operator1/1 -> Unit Delay1/1
  Constant3/1 -> Relational Operator1/2
  Discrete-Time Integrator1/1 -> ramp_out/1, Relational Operator1/1
  fc/1 -> Discrete-Time Integrator1/1

== system TestAsset14/Choppe Control1/Pulse Generator ==
  Duty_Cycle : Inport
  Add : Sum  Inputs=-+
  Constant3 : Constant
  Constant4 : Constant  Value=0
  Digital Clock : DigitalClock  SampleTime=Ts
  Divide2 : Product  Inputs=**
  Divide3 : Product  Inputs=**
  Math Function : Math  Operator=mod  SaturateOnIntegerOverflow=on
  Nb_of_samples_by_cycle : Constant  Value=1/Freq_sawtooth/Ts
  Relational Operator1 : RelationalOperator  Operator=>  OutDataTypeStr=boolean  RndMeth=Nearest
  Rounding Function1 : Rounding  Operator=round
  Switch : Switch  Threshold=0.5
  Ts : Constant  Value=Ts
  Pulse : Outport
  wires:
  Math Function/1 -> Relational Operator1/2
  Constant4/1 -> Switch/3
  Constant3/1 -> Switch/1
  Relational Operator1/1 -> Switch/2
  Nb_of_samples_by_cycle/1 -> Rounding Function1/1
  Divide2/1 -> Relational Operator1/1
  Divide3/1 -> Add/2, Math Function/2  "Period_of_cycle"
  Duty_Cycle/1 -> Divide2/1
  Rounding Function1/1 -> Divide3/2  "Nb_of_samples_by_cycle"
  Ts/1 -> Divide3/1, Add/1
  Digital Clock/1 -> Math Function/1
  Add/1 -> Divide2/2
  Switch/1 -> Pulse/1

== system TestAsset14/G state/Switch2 ==
  Vdq : Inport
  Compare To Constant1 : simulink/Logic and Bit Operations/Compare To Constant  relop=<  const=388  OutDataTypeStr=boolean
  Fcn1 : Fcn  Expr=sqrt(u(1)^2+u(2)^2)
  Scope2 : Scope
  SW : Outport
  wires:
  Vdq/1 -> Fcn1/1
  Fcn1/1 -> Scope2/1, Compare To Constant1/1
  Compare To Constant1/1 -> SW/1

== system TestAsset14/Generator side control1/Discrete SV PWM Generator ==
  note: Space Vector Pulse Width Modulation (SV PWM)
  note: Pierre Giroux, Gilbert Sybille
      | Power System Laboratory, IREQ
      | Hydro-Quebec
  note: Hoang Le-Huy
      | Universite Laval
      | Quebec
  Ualpha : Inport
  Ubeta : Inport  Port=2
  Constant : Constant
  Constant1 : Constant  Value=Freq
  Constant2 : Constant  Value=m
  Constant3 : Constant  Value=Pha
  Constant4 : Constant  Value=SwitchingPattern
  Determine reference vector (U*) : Subsystem
  INFO : Subsystem
      mask Display: disp('?')
  Logical Operator : Logic  Operator=NOT  AllPortsSameDT=off
  Multiport Switch : MultiPortSwitch  Inputs=2  SaturateOnIntegerOverflow=on
  Relational Operator : RelationalOperator  Operator===  RndMeth=Nearest
  SV Modulator Pattern #1 : Subsystem
  SV Modulator Pattern #2 : Subsystem
  Pulses : Outport
  wires:
  Ualpha/1 -> Determine reference vector (U*)/1(In1)
  Ubeta/1 -> Determine reference vector (U*)/2(In2)
  SV Modulator Pattern #1/1(Pulses) -> Multiport Switch/2
  SV Modulator Pattern #2/1(Pulses) -> Multiport Switch/3
  Multiport Switch/1 -> Pulses/1
  Determine reference vector (U*)/1(m) -> SV Modulator Pattern #2/1(m), SV Modulator Pattern #1/1(m)
  Determine reference vector (U*)/2(alpha) -> SV Modulator Pattern #2/2(alpha), SV Modulator Pattern #1/2(alpha)
  Constant2/1 -> Determine reference vector (U*)/3(m_Int)
  Constant1/1 -> Determine reference vector (U*)/4(Freq_Int)
  Constant3/1 -> Determine reference vector (U*)/5(Pha_Init)
  Constant4/1 -> Multiport Switch/1, Relational Operator/1
  Constant/1 -> Relational Operator/2
  Relational Operator/1 -> SV Modulator Pattern #1/Enable, Logical Operator/1
  Logical Operator/1 -> SV Modulator Pattern #2/Enable

== system TestAsset14/Generator side control1/PI  for Isd ==
  note: Discrete PID Controller
  note: Pierre Giroux, Gilbert Sybille
      | Power System Simulation Laboratory
      | IREQ, Hydro-Quebc
  Error : Inport  SampleTime=Ts
  Discrete-Time Integrator : DiscreteIntegrator  InitialCondition=Init  SampleTime=Ts  UpperSaturationLimit=UpperLimit  LowerSaturationLimit=LowerLimit  ICPrevOutput=DiscIntNeverNeededParam  ICPrevScaledInput=DiscIntNeverNeededParam
  Kp4 : Gain  Gain=Kp  SaturateOnIntegerOverflow=on  SampleTime=Ts  OutDataTypeStr=Inherit: Same as input  ParamDataTypeStr=Inherit: Same as input
  Kp5 : Gain  Gain=Ki  SaturateOnIntegerOverflow=on  SampleTime=Ts  OutDataTypeStr=Inherit: Same as input  ParamDataTypeStr=Inherit: Same as input
  Saturation2 : Saturate  UpperLimit=UpperLimit  LowerLimit=LowerLimit  SampleTime=Ts
  Sum6 : Sum  InputSameDT=on  SaturateOnIntegerOverflow=on  SampleTime=Ts  OutDataTypeStr=Inherit: Same as first input
  Zero-Order Hold : ZeroOrderHold  SampleTime=Ts
  Out : Outport  SampleTime=Ts  InitialOutput=0
  wires:
  Zero-Order Hold/1 -> Sum6/1
  Saturation2/1 -> Out/1
  Discrete-Time Integrator/1 -> Sum6/2
  Kp4/1 -> Zero-Order Hold/1
  Kp5/1 -> Discrete-Time Integrator/1
  Sum6/1 -> Saturation2/1
  Error/1 -> Kp5/1, Kp4/1

== system TestAsset14/Generator side control1/PI  for Isq ==
  note: Pierre Giroux, Gilbert Sybille
      | Power System Simulation Laboratory
      | IREQ, Hydro-Quebc
  note: Discrete PID Controller
  Error : Inport  SampleTime=Ts
  Discrete-Time Integrator : DiscreteIntegrator  InitialCondition=Init  SampleTime=Ts  UpperSaturationLimit=UpperLimit  LowerSaturationLimit=LowerLimit  ICPrevOutput=DiscIntNeverNeededParam  ICPrevScaledInput=DiscIntNeverNeededParam
  Kp4 : Gain  Gain=Kp  SaturateOnIntegerOverflow=on  SampleTime=Ts  OutDataTypeStr=Inherit: Same as input  ParamDataTypeStr=Inherit: Same as input
  Kp5 : Gain  Gain=Ki  SaturateOnIntegerOverflow=on  SampleTime=Ts  OutDataTypeStr=Inherit: Same as input  ParamDataTypeStr=Inherit: Same as input
  Saturation2 : Saturate  UpperLimit=UpperLimit  LowerLimit=LowerLimit  SampleTime=Ts
  Sum6 : Sum  InputSameDT=on  SaturateOnIntegerOverflow=on  SampleTime=Ts  OutDataTypeStr=Inherit: Same as first input
  Zero-Order Hold : ZeroOrderHold  SampleTime=Ts
  Out : Outport  SampleTime=Ts  InitialOutput=0
  wires:
  Error/1 -> Kp4/1, Kp5/1
  Sum6/1 -> Saturation2/1
  Kp5/1 -> Discrete-Time Integrator/1
  Kp4/1 -> Zero-Order Hold/1
  Discrete-Time Integrator/1 -> Sum6/2
  Saturation2/1 -> Out/1
  Zero-Order Hold/1 -> Sum6/1

== system TestAsset14/Generator side control1/Speed & Pitch Control ==
  note: Speed Regulator
  note: P
  note: Te_ref
  note: pu_mec->
  wr(pu) : Inport
  Te(pu) : Inport  Port=2
  0-inf : Saturate  UpperLimit=inf  LowerLimit=0  SampleTime=20e-6
  1-D Lookup Table : Lookup_n-D  NumberOfTableDimensions=1  BreakpointsForDimension1=[0,0.1,0.18,0.29,0.415,0.515,0.8,1.075]  Table=[0,0.5,0.62,0.71,0.81,0.91,1.025, 1.11]  SampleTime=20e-6  RndMeth=Simplest  InputSameDT=on
  Discrete PI Controller : powerlib_extras/Discrete  Control Blocks/Discrete PI Controller  Kp=0.3  Ki=0.1  Par_Limits=[inf 0]  Init=0.9  Ts=20e-6
  Discrete 2nd-Order Filter3 : powerlib_extras/Discrete  Control Blocks/Discrete  2nd-Order Filter  FilterType=Lowpass  Fo=2  Zeta=0.6  Ts=20e-6  Initialize=on  Vac_Init=[0 0 0]  Vdc_Init=-100  PlotResponse=off  param1=[1 500 1]
  Gain1 : Gain  Gain=-2/(3*14*1)  SaturateOnIntegerOverflow=on  OutDataTypeStr=Inherit: Same as input  ParamDataTypeStr=Inherit: Same as input
  Gain3 : Gain  Gain=300e3/0.9/(2*pi*60/14)  SaturateOnIntegerOverflow=on  OutDataTypeStr=Inherit: Same as input  ParamDataTypeStr=Inherit: Same as input
  Product : Product  RndMeth=Zero
  Scope1 : Scope
  Scope2 : Scope  NumInputPorts=2
  Scope3 : Scope
  Scope4 : Scope
  Sum1 : Sum  Inputs=-|+
  Switch : Switch  Threshold=0.75
  pu_elec->pu_mec : Gain  Gain=1/0.9  SampleTime=20e-6
  wref : Constant
  Iq_ref : Outport
  tag scope: wr_pu=global
  wires:
  wr(pu)/1 -> Sum1/2, Product/2, [wr_pu]  "wr"
  0-inf/1 -> Scope4/1, pu_elec->pu_mec/1
  pu_elec->pu_mec/1 -> 1-D Lookup Table/1, Switch/2  "Pmes"
  wref/1 -> Switch/1
  Switch/1 -> Scope3/1, Sum1/1  "wref"
  Sum1/1 -> Discrete PI Controller/1
  1-D Lookup Table/1 -> Switch/3
  Product/1 -> 0-inf/1
  Te(pu)/1 -> Product/1
  Discrete PI Controller/1 -> Scope1/1, Gain3/1
  Discrete 2nd-Order Filter3/1 -> Scope2/2, Iq_ref/1
  Gain1/1 -> Scope2/1, Discrete 2nd-Order Filter3/1
  Gain3/1 -> Gain1/1

== system TestAsset14/Grid side control/Discrete PI Controller1 ==
  note: Pierre Giroux, Gilbert Sybille
      | Power System Simulation Laboratory
      | IREQ, Hydro-Quebc
  note: Discrete PID Controller
  Error : Inport  SampleTime=Ts
  Discrete-Time Integrator : DiscreteIntegrator  InitialCondition=Init  SampleTime=Ts  LimitOutput=on  UpperSaturationLimit=UpperLimit  LowerSaturationLimit=LowerLimit  ICPrevOutput=DiscIntNeverNeededParam  ICPrevScaledInput=DiscIntNeverNeededParam
  Kp4 : Gain  Gain=Kp  SaturateOnIntegerOverflow=on  SampleTime=Ts  OutDataTypeStr=Inherit: Same as input  ParamDataTypeStr=Inherit: Same as input
  Kp5 : Gain  Gain=Ki  SaturateOnIntegerOverflow=on  SampleTime=Ts  OutDataTypeStr=Inherit: Same as input  ParamDataTypeStr=Inherit: Same as input
  Saturation2 : Saturate  UpperLimit=UpperLimit  LowerLimit=LowerLimit  SampleTime=Ts
  Sum6 : Sum  InputSameDT=on  SaturateOnIntegerOverflow=on  SampleTime=Ts  OutDataTypeStr=Inherit: Same as first input
  Zero-Order Hold : ZeroOrderHold  SampleTime=Ts
  Out : Outport  SampleTime=Ts  InitialOutput=0
  wires:
  Error/1 -> Kp4/1, Kp5/1
  Sum6/1 -> Saturation2/1
  Kp5/1 -> Discrete-Time Integrator/1
  Kp4/1 -> Zero-Order Hold/1
  Discrete-Time Integrator/1 -> Sum6/2
  Saturation2/1 -> Out/1
  Zero-Order Hold/1 -> Sum6/1

== system TestAsset14/Grid side control/Discrete PI Controller2 ==
  note: Discrete PID Controller
  note: Pierre Giroux, Gilbert Sybille
      | Power System Simulation Laboratory
      | IREQ, Hydro-Quebc
  Error : Inport  SampleTime=Ts
  Discrete-Time Integrator : DiscreteIntegrator  InitialCondition=Init  SampleTime=Ts  LimitOutput=on  UpperSaturationLimit=UpperLimit  LowerSaturationLimit=LowerLimit  ICPrevOutput=DiscIntNeverNeededParam  ICPrevScaledInput=DiscIntNeverNeededParam
  Kp4 : Gain  Gain=Kp  SaturateOnIntegerOverflow=on  SampleTime=Ts  OutDataTypeStr=Inherit: Same as input  ParamDataTypeStr=Inherit: Same as input
  Kp5 : Gain  Gain=Ki  SaturateOnIntegerOverflow=on  SampleTime=Ts  OutDataTypeStr=Inherit: Same as input  ParamDataTypeStr=Inherit: Same as input
  Saturation2 : Saturate  UpperLimit=UpperLimit  LowerLimit=LowerLimit  SampleTime=Ts
  Sum6 : Sum  InputSameDT=on  SaturateOnIntegerOverflow=on  SampleTime=Ts  OutDataTypeStr=Inherit: Same as first input
  Zero-Order Hold : ZeroOrderHold  SampleTime=Ts
  Out : Outport  SampleTime=Ts  InitialOutput=0
  wires:
  Zero-Order Hold/1 -> Sum6/1
  Saturation2/1 -> Out/1
  Discrete-Time Integrator/1 -> Sum6/2
  Kp4/1 -> Zero-Order Hold/1
  Kp5/1 -> Discrete-Time Integrator/1
  Sum6/1 -> Saturation2/1
  Error/1 -> Kp5/1, Kp4/1

== system TestAsset14/Grid side control/Discrete PI Controller3 ==
  note: Pierre Giroux, Gilbert Sybille
      | Power System Simulation Laboratory
      | IREQ, Hydro-Quebc
  note: Discrete PID Controller
  Error : Inport  SampleTime=Ts
  Discrete-Time Integrator : DiscreteIntegrator  InitialCondition=Init  SampleTime=Ts  LimitOutput=on  UpperSaturationLimit=UpperLimit  LowerSaturationLimit=LowerLimit  ICPrevOutput=DiscIntNeverNeededParam  ICPrevScaledInput=DiscIntNeverNeededParam
  Kp4 : Gain  Gain=Kp  SaturateOnIntegerOverflow=on  SampleTime=Ts  OutDataTypeStr=Inherit: Same as input  ParamDataTypeStr=Inherit: Same as input
  Kp5 : Gain  Gain=Ki  SaturateOnIntegerOverflow=on  SampleTime=Ts  OutDataTypeStr=Inherit: Same as input  ParamDataTypeStr=Inherit: Same as input
  Saturation2 : Saturate  UpperLimit=UpperLimit  LowerLimit=LowerLimit  SampleTime=Ts
  Sum6 : Sum  InputSameDT=on  SaturateOnIntegerOverflow=on  SampleTime=Ts  OutDataTypeStr=Inherit: Same as first input
  Zero-Order Hold : ZeroOrderHold  SampleTime=Ts
  Out : Outport  SampleTime=Ts  InitialOutput=0
  wires:
  Error/1 -> Kp4/1, Kp5/1
  Sum6/1 -> Saturation2/1
  Kp5/1 -> Discrete-Time Integrator/1
  Kp4/1 -> Zero-Order Hold/1
  Discrete-Time Integrator/1 -> Sum6/2
  Saturation2/1 -> Out/1
  Zero-Order Hold/1 -> Sum6/1

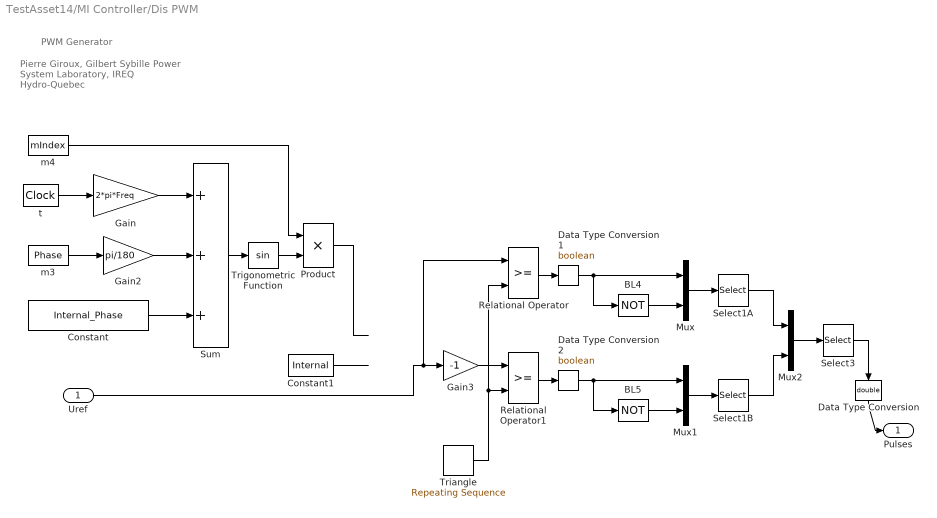
== system TestAsset14/MI Controller/Dis PWM ==
  note: Pierre Giroux, Gilbert Sybille
      | Power System Laboratory, IREQ
      | Hydro-Quebec
  note: PWM Generator
  Uref : Inport
  BL4 : Logic  Operator=NOT  Inputs=1
  BL5 : Logic  Operator=NOT  Inputs=1
  Constant : Constant  Value=Internal_Phase
  Constant1 : Constant  Value=Internal
  Data Type Conversion : DataTypeConversion  OutDataTypeStr=double  SaturateOnIntegerOverflow=on  RndMeth=Zero
  Data Type Conversion1 : DataTypeConversion  OutDataTypeStr=boolean  SaturateOnIntegerOverflow=on  RndMeth=Zero
  Data Type Conversion2 : DataTypeConversion  OutDataTypeStr=boolean  SaturateOnIntegerOverflow=on  RndMeth=Zero
  Gain : Gain  Gain=2*pi*Freq  SaturateOnIntegerOverflow=on  OutDataTypeStr=Inherit: Same as input  ParamDataTypeStr=Inherit: Same as input
  Gain2 : Gain  Gain=pi/180  SaturateOnIntegerOverflow=on  OutDataTypeStr=Inherit: Same as input  ParamDataTypeStr=Inherit: Same as input
  Gain3 : Gain  Gain=-1  SaturateOnIntegerOverflow=on  OutDataTypeStr=Inherit: Same as input  ParamDataTypeStr=Inherit: Same as input
  Mux : Mux  Inputs=2
  Mux1 : Mux  Inputs=2
  Mux2 : Mux  Inputs=2
  Product : Product  InputSameDT=on  SaturateOnIntegerOverflow=on  OutDataTypeStr=Inherit: Same as first input
  Relational Operator : RelationalOperator  RndMeth=Nearest  InputSameDT=on
  Relational Operator1 : RelationalOperator  RndMeth=Nearest  InputSameDT=on
  Select1A : Selector  InputPortWidth=Select1_PortWidth  IndexOptions=Index vector (dialog)  Indices=Select1_Elements  OutputSizes=1
  Select1B : Selector  InputPortWidth=Select1_PortWidth  IndexOptions=Index vector (dialog)  Indices=Select1_Elements  OutputSizes=1
  Select3 : Selector  InputPortWidth=Select3_PortWidth  IndexOptions=Index vector (dialog)  Indices=Select3_Elements  OutputSizes=1
  Sum : Sum  Inputs=+++  InputSameDT=on  SaturateOnIntegerOverflow=on  OutDataTypeStr=Inherit: Same as first input
  Triangle : simulink/Sources/Repeating Sequence  rep_seq_t=[0 1/Fc/4 3/Fc/4 1/Fc]  rep_seq_y=[0 -1 1 0]
  Trigonometric Function : Trigonometry
  m3 : Constant  Value=Phase
  m4 : Constant  Value=mIndex
  t : DigitalClock  SampleTime=Ts
  Pulses : Outport
  wires:
  Mux2/1 -> Select3/1
  Select1B/1 -> Mux2/2
  Select1A/1 -> Mux2/1
  Mux1/1 -> Select1B/1
  Mux/1 -> Select1A/1
  BL5/1 -> Mux1/2
  BL4/1 -> Mux/2
  Gain3/1 -> Relational Operator1/1
  Triangle/1 -> Relational Operator1/2, Relational Operator/2
  Product/1 -> ?
  Constant1/1 -> ?
  Uref/1 -> Relational Operator/1, Gain3/1
  Trigonometric Function/1 -> Product/2
  Sum/1 -> Trigonometric Function/1
  m4/1 -> Product/1
  Constant/1 -> Sum/3
  m3/1 -> Gain2/1
  Gain2/1 -> Sum/2
  Gain/1 -> Sum/1
  t/1 -> Gain/1
  Select3/1 -> Data Type Conversion/1
  Data Type Conversion/1 -> Pulses/1
  Relational Operator/1 -> Data Type Conversion1/1
  Data Type Conversion1/1 -> BL4/1, Mux/1
  Relational Operator1/1 -> Data Type Conversion2/1
  Data Type Conversion2/1 -> BL5/1, Mux1/1

== system TestAsset14/MI Controller/Switch2 ==
  Vdq : Inport
  Compare To Constant1 : simulink/Logic and Bit Operations/Compare To Constant  relop=<  const=388  OutDataTypeStr=boolean
  Fcn1 : Fcn  Expr=sqrt(u(1)^2+u(2)^2)
  SW : Outport
  wires:
  Vdq/1 -> Fcn1/1
  Fcn1/1 -> Compare To Constant1/1
  Compare To Constant1/1 -> SW/1

== system TestAsset14/MI Controller/central control ==
  Vdq_load : Inport
  Vdq_droop : Inport  Port=2
  Add1 : Sum
  Add2 : Sum
  Demux1 : Demux  Outputs=2
  Demux2 : Demux  Outputs=2
  Discrete PI Controller1 : powerlib_extras/Discrete  Control Blocks/Discrete PI Controller  Kp=0.2  Ki=40  Par_Limits=[100 -100]  Init=0  Ts=2e-05
  Discrete PI Controller2 : powerlib_extras/Discrete  Control Blocks/Discrete PI Controller  Kp=0.2  Ki=40  Par_Limits=[100 -100]  Init=0  Ts=2e-05
  Mux4 : Mux  Inputs=2
  Sum1 : Sum  Inputs=-+
  Sum2 : Sum  Inputs=-+
  v1 : Scope  NumInputPorts=2
  v5 : Scope  NumInputPorts=2
  out : Outport
  wires:
  Mux4/1 -> out/1
  Vdq_load/1 -> v1/1, Demux2/1
  Vdq_droop/1 -> v1/2, Demux1/1
  Demux2/1 -> Sum1/1
  Demux2/2 -> Sum2/1
  Sum1/1 -> Discrete PI Controller2/1
  Sum2/1 -> Discrete PI Controller1/1
  Demux1/2 -> Add2/2, Sum2/2
  Discrete PI Controller1/1 -> v5/2, Add2/1
  Discrete PI Controller2/1 -> v5/1, Add1/1
  Demux1/1 -> Add1/2, Sum1/2
  Add1/1 -> Mux4/1
  Add2/1 -> Mux4/2

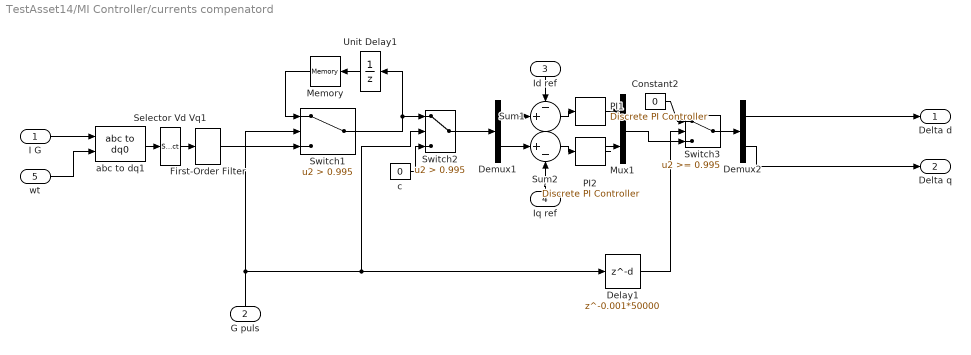
== system TestAsset14/MI Controller/currents compenatord ==
  I G : Inport
  G puls : Inport  Port=2
  Id ref : Inport  Port=3
  Iq ref : Inport  Port=4
  wt : Inport  Port=5
  Constant2 : Constant  Value=0
  Delay1 : Delay  DelayLength=0.001*50000  InitialCondition=0  SampleTime=2e-05
  Demux1 : Demux  Outputs=2
  Demux2 : Demux  Outputs=2
  First-Order Filter : powerlib_meascontrol/Filters/First-Order Filter  FilterType=Lowpass  Tc=1e-3  Ts=0  Initialize=on  Vac_Init=[0, 0, 50]  Vdc_Init=0  PlotResponse=off  FreqRange="[0,  200,  1]"
  Memory : Memory
  Mux1 : Mux  Inputs=2
  "PI1 " : powerlib_extras/Discrete  Control Blocks/Discrete PI Controller  Kp=0.1  Ki=4  Par_Limits=[200 -200]  Init=0  Ts=2e-05
  PI2 : powerlib_extras/Discrete  Control Blocks/Discrete PI Controller  Kp=0.1  Ki=4  Par_Limits=[200 -200]  Init=0  Ts=2e-05
  Selector Vd Vq1 : Selector  InputPortWidth=3  IndexOptions=Index vector (dialog)  Indices=[1 2]  OutputSizes=1
  Sum1 : Sum  Inputs=-+|
  Sum2 : Sum  Inputs=|+-
  Switch1 : Switch  Criteria=u2 > Threshold  Threshold=0.995
  Switch2 : Switch  Criteria=u2 > Threshold  Threshold=0.995
  Switch3 : Switch  Threshold=0.995
  Unit Delay1 : UnitDelay  SampleTime=2e-05  HasFrameUpgradeWarning=on
  abc to dq1 : powerlib_meascontrol/Transformations/abc to dq0  Alignment=90 degrees behind phase A axis
  c : Constant  Value=0
  Delta d : Outport
  Delta q : Outport  Port=2
  wires:
  wt/1 -> abc to dq1/2
  Iq ref/1 -> Sum2/2
  Id ref/1 -> Sum1/1
  I G/1 -> abc to dq1/1
  abc to dq1/1 -> Selector Vd Vq1/1
  First-Order Filter/1 -> Switch1/3
  Switch1/1 -> Switch2/1, Unit Delay1/1
  Memory/1 -> Switch1/1
  Unit Delay1/1 -> Memory/1
  Demux1/1 -> Sum1/2
  Demux1/2 -> Sum2/1
  Sum2/1 -> PI2/1
  Sum1/1 -> "PI1 "/1
  Mux1/1 -> Switch3/3
  Demux2/1 -> Delta d/1
  Demux2/2 -> Delta q/1
  Switch3/1 -> Demux2/1
  Constant2/1 -> Switch3/1
  G puls/1 -> Switch2/2, Delay1/1, Switch1/2
  Selector Vd Vq1/1 -> First-Order Filter/1
  Delay1/1 -> Switch3/2
  "PI1 "/1 -> Mux1/1
  PI2/1 -> Mux1/2
  Switch2/1 -> Demux1/1
  c/1 -> Switch2/3
